simulink library "NeuroMuscularLibrary"  (R2019b)
settings: Solver=ode45  StartTime=0.0  StopTime=10.0  RelTol=1e-3  EnableMultiTasking=on
values from neighbouring files (symbols this model uses):
  a_18_19 = 116    [Prosthesis3R60Params.m]
  a_18_21 = 34    [Prosthesis3R60Params.m]
  a_2_3 = 18    [Prosthesis3R60Params.m]
  angle_offset = 0    [Prosthesis3R60Params.m]
  ankle_height = 0.08    [BodyMechParams.m]
  c = 0.05    [BodyMechParams.m]
  c_jointstop = 0.3 / (pi/180)    (= 17.1887338539)    [BodyMechParams.m]
  c_stance_comp_a0 = 885.0653    [Prosthesis3R60Params.m]
  c_stance_comp_a1 = 2.1443    [Prosthesis3R60Params.m]
  cg14 = 1/2*L14    (= 0.0475)    [Prosthesis3R60Params.m]
  cg25 = (5.45/11.05)*L25    (= 0.0379527149321)    [Prosthesis3R60Params.m]
  cg3 = (3.6/10.4)*L3    (= 0.0306346153846)    [Prosthesis3R60Params.m]
  d_fBall = 0.1    [BodyMechParams.m]
  d_fHeel = 0.05    [BodyMechParams.m]
  deltaLegAngleThr = 8*pi/180    (= 0.13962634016)    [CMGParams.m]
  DeltaThRef = 2e-3    (= 0.002)    [BodyMechParams.m]
  dt_visual = 0.001    [Prosthesis3R60Params.m]
  eref = 0.04    [BodyMechParams.m]
  Fmax = 4000    [MuscleEnergyTest.m]
  FmaxGLU = 1500    [BodyMechParams.m]
  footBallToAnkleDist = 0.16    [BodyMechParams.m]
  footBallToCenterDist = footLength/2    (= 0.1)    [BodyMechParams.m]
  footBallToHeelDist = footLength    (= 0.2)    [BodyMechParams.m]
  footCenterToCGDist = 0.14 - footBallToCenterDist    (= 0.04)    [BodyMechParams.m]
  footInertia = 0.005    [BodyMechParams.m]
  footLength = 0.2    [BodyMechParams.m]
  footMass = 1.25    [BodyMechParams.m]
  FT = 20    [MuscleEnergyTest.m]
  FT_GLU = 47.6    [BodyMechParams.m]
  g = 9.80665    [BodyMechParams.m]
  groundTheta = [atan(diff(groundZ)./diff(groundX)), 0]    [generateGround.m]
  groundZ = groundZ * stepSize/(largestStep+eps)    [generateGround.m]
  hatCenterToCGDist = 0.35 - hatHipToCenterDistLen    (= -0.05)    [BodyMechParams.m]
  hatHipToCenterDistLen = hatLength/2    (= 0.4)    [BodyMechParams.m]
  hatInertia = 3    [BodyMechParams.m]
  hatLeftHipToCenterDistWidth = .15    (= 0.15)    [BodyMechParams.m]
  hatLength = 0.8    [BodyMechParams.m]
  hatMass = 53.5    [BodyMechParams.m]
  hatThickness = 0.2    [BodyMechParams.m]
  hatWidth = 0.4    [BodyMechParams.m]
  J1011 = (4130)*1e-9    (= 4.13e-06)    [Prosthesis3R60Params.m]
  J1415 = (1.18*1e5)*1e-9    (= 0.000118)    [Prosthesis3R60Params.m]
  J18192021 = (6.86*1e4)*1e-9    (= 6.86e-05)    [Prosthesis3R60Params.m]
  J2526 = (3.59*1e4)*1e-9    (= 3.59e-05)    [Prosthesis3R60Params.m]
  J3467 = (25.96*1e4)*1e-9    (= 0.0002596)    [Prosthesis3R60Params.m]
  K = 5    [BodyMechParams.m]
  k_gn = k_gn/2    (= 39226.6)    [BodyMechParams.m]
  k_gt = k_gt/2    (= 39226.6)    [BodyMechParams.m]
  k_pressure = hatMass * g / DeltaThRef    (= 262327.8875)    [BodyMechParams.m]
  k_stance = 130000    [Prosthesis3R60Params.m]
  k_swing = 18750    [Prosthesis3R60Params.m]
  L0_stance = 0.08925    [Prosthesis3R60Params.m]
  L0_swing = 0.0896    [Prosthesis3R60Params.m]
  L10 = 7.9*1e-3    (= 0.0079)    [Prosthesis3R60Params.m]
  L11 = 3.3*1e-3    (= 0.0033)    [Prosthesis3R60Params.m]
  L14 = 95*1e-3    (= 0.095)    [Prosthesis3R60Params.m]
  L15 = 8.2*1e-3    (= 0.0082)    [Prosthesis3R60Params.m]
  L18 = 25.1*1e-3    (= 0.0251)    [Prosthesis3R60Params.m]
  L19 = 17.7*1e-3    (= 0.0177)    [Prosthesis3R60Params.m]
  L20 = 26*1e-3    (= 0.026)    [Prosthesis3R60Params.m]
  L21 = 1.7*1e-3    (= 0.0017)    [Prosthesis3R60Params.m]
  L25 = 76.95*1e-3    (= 0.07695)    [Prosthesis3R60Params.m]
  L26 = 2.8*1e-3    (= 0.0028)    [Prosthesis3R60Params.m]
  L3 = 88.5*1e-3    (= 0.0885)    [Prosthesis3R60Params.m]
  L4 = 1.7*1e-3    (= 0.0017)    [Prosthesis3R60Params.m]
  L6 = 40.25*1e-3    (= 0.04025)    [Prosthesis3R60Params.m]
  L7 = 14.9*1e-3    (= 0.0149)    [Prosthesis3R60Params.m]
  leg_l = [(thighLength - ankle_height/2) (shankLength - ankle_height/2)]    [BodyMechParams.m]
  legAngleSpeedMax = 10    [CMGParams.m]
  lopt = 0.055    [MuscleEnergyTest.m]
  loptBFSH = 0.12    [BodyMechParams.m]
  loptGAS = 0.05    [BodyMechParams.m]
  loptGLU = 0.11    [BodyMechParams.m]
  loptHAB = 0.09    [BodyMechParams.m]
  loptHAD = 0.10    (= 0.1)    [BodyMechParams.m]
  loptHAM = 0.10    (= 0.1)    [BodyMechParams.m]
  loptHFL = 0.11    [BodyMechParams.m]
  loptRF = 0.08    [BodyMechParams.m]
  loptSOL = 0.04    [BodyMechParams.m]
  loptTA = 0.06    [BodyMechParams.m]
  loptVAS = 0.08    [BodyMechParams.m]
  lslack = 0.245    [MuscleEnergyTest.m]
  lslackBFSH = 0.10    (= 0.1)    [BodyMechParams.m]
  lslackGAS = 0.40    (= 0.4)    [BodyMechParams.m]
  lslackGLU = 0.13    [BodyMechParams.m]
  lslackHAB = 0.07    [BodyMechParams.m]
  lslackHAD = 0.18    [BodyMechParams.m]
  lslackHAM = 0.31    [BodyMechParams.m]
  lslackHFL = 0.10    (= 0.1)    [BodyMechParams.m]
  lslackRF = 0.35    [BodyMechParams.m]
  lslackSOL = 0.26    [BodyMechParams.m]
  lslackTA = 0.24    [BodyMechParams.m]
  lslackVAS = 0.23    [BodyMechParams.m]
  m1011 = 49.5*1e-3    (= 0.0495)    [Prosthesis3R60Params.m]
  m1415 = 123.8*1e-3    (= 0.1238)    [Prosthesis3R60Params.m]
  m18192021 = 196.6*1e-3    (= 0.1966)    [Prosthesis3R60Params.m]
  m2526 = 58.3*1e-3    (= 0.0583)    [Prosthesis3R60Params.m]
  m3467 = 253.3*1e-3    (= 0.2533)    [Prosthesis3R60Params.m]
  mu_slide = 0.8    [BodyMechParams.m]
  mu_stick = 0.9    [BodyMechParams.m]
  N = 1.5    [BodyMechParams.m]    (also in cmaes.m = size(x,1); mergeCompareEnergyCosts.m = {S.name})
  phiKneeUpLimit = 5*pi/180    (= 0.0872664625997)    [BodyMechParams.m]
  phimaxGASa = (100-90)*pi/180    (= 0.174532925199)    [BodyMechParams.m]
  phimaxGASk = (180-140)*pi/180    (= 0.698131700798)    [BodyMechParams.m]
  phimaxRFk = (180-165)*pi/180    (= 0.261799387799)    [BodyMechParams.m]
  phimaxSOL = (100-90)*pi/180    (= 0.174532925199)    [BodyMechParams.m]
  phimaxTA = (80-90)*pi/180    (= -0.174532925199)    [BodyMechParams.m]
  phimaxVAS = (180-165)*pi/180    (= 0.261799387799)    [BodyMechParams.m]
  phirefBFSH = (180-160)*pi/180    (= 0.349065850399)    [BodyMechParams.m]
  phirefGASa = (80-90)*pi/180    (= -0.174532925199)    [BodyMechParams.m]
  phirefGASk = (180-165)*pi/180    (= 0.261799387799)    [BodyMechParams.m]
  phirefGLU = (120-180)*pi/180    (= -1.0471975512)    [BodyMechParams.m]
  phirefHAB = 10*pi/180    (= 0.174532925199)    [BodyMechParams.m]
  phirefHAD = 15*pi/180    (= 0.261799387799)    [BodyMechParams.m]
  phirefHAMh = (150-180)*pi/180    (= -0.523598775598)    [BodyMechParams.m]
  phirefHAMk = (180-180)*pi/180    (= 0)    [BodyMechParams.m]
  phirefHFL = (160-180)*pi/180    (= -0.349065850399)    [BodyMechParams.m]
  phirefRFh = (170-180)*pi/180    (= -0.174532925199)    [BodyMechParams.m]
  phirefRFk = (180-125)*pi/180    (= 0.959931088597)    [BodyMechParams.m]
  phirefSOL = (90-90)*pi/180    (= 0)    [BodyMechParams.m]
  ... (+64 more)
undefined symbols (not defined in the file or in its folder): ankleBackDriveGain, ankleCJointstop, ankleDgain, ankleFilterPID, ankleFilterSEA, ankleGearEff, ankleGearRatio, ankleIgain, ankleInitialAngle, ankleInputMass, ankleIntCoulomb, ankleIntDamping, ankleIntStatic, ankleParallelSpringDamping, ankleParallelSpringOffset, ankleParallelSpringStiffness, anklePgain, anklePlantarLimit, ankleSEADamping, ankleSEAStiffness, ankleTendonMass, ankleWMaxJointstop, D12_F, D12_S, D12_T, D12z_T, D13_F, D1G_F, D1G_HAT, D1G_S, D1G_T, D1Gy_F, DeltaS, DeltaSGLU, DeltaSHFL, dryFrictionDamping, dryFrictionStiffness, dryFrictionVelThresh, footMassp, FourBarL1, FourBarL3, GainDphiHATGLUst, GainDphiHATHABst, GainDphiHATHADst, GainDphiHATHFLst, GainFGASst, GainFGLUst, GainFHABst, GainFHAMst, GainFSOLst, GainFSOLTAst, GainFVASst, GainGAS, GainGLU, GainGLUswing, GainHAM, GainHAMHFL ... (+194)
libraries: sm_lib x332, nesl_utility x156, simulink x33, dspswit3 x30, $bdroot x19, simulink_extras x7
(part 1 of 15)
settings Model: Creator=nitisht  LastModifiedBy=Nathan
settings DataIOCC: LimitDataPoints=on  SaveFormat=Array  ReturnWorkspaceOutputs=off
settings OptimizationCC: LifeSpan=inf
settings DebuggingCC: UnderspecifiedInitializationDetection=Classic  MergeDetectMultiDrivingBlocksExec=none  SolverPrmCheckMsg=warning  StateNameClashWarn=warning  SFUnexpectedBacktrackingDiag=warning  SFNoUnconditionalDefaultTransitionDiag=warning  SFExecutionAtInitializationDiag=none  ArithmeticOperatorsInVariantConditions=warning
settings HardwareCC: ProdBitPerLong=64  ProdLargestAtomicFloat=None  ProdIntDivRoundTo=Undefined  ProdEndianess=Unspecified  ProdHWDeviceType=Intel->x86-64
settings ModelReferenceCC: PropagateSignalLabelsOutOfModel=off
settings SFSimCC: SimUseLocalCustomCode=off  CustomCodeUndefinedFunction=UseInterfaceOnly
settings RTWCC: RTWUseLocalCustomCode=off  RTWCompilerOptimization=on
settings CodeAppCC: StateflowObjectComments=on
settings GRTTargetCC: TargetLangStandard=C89/C90 (ANSI)  GeneratePreprocessorConditionals=Disable all
settings ConfigComp: CovMetricSettings=dw  CovHtmlReporting=on  CovSaveCumulativeToWorkspaceVar=on  CovSaveSingleToWorkspaceVar=on  CovExternalEMLEnable=off  CovSFcnEnable=off

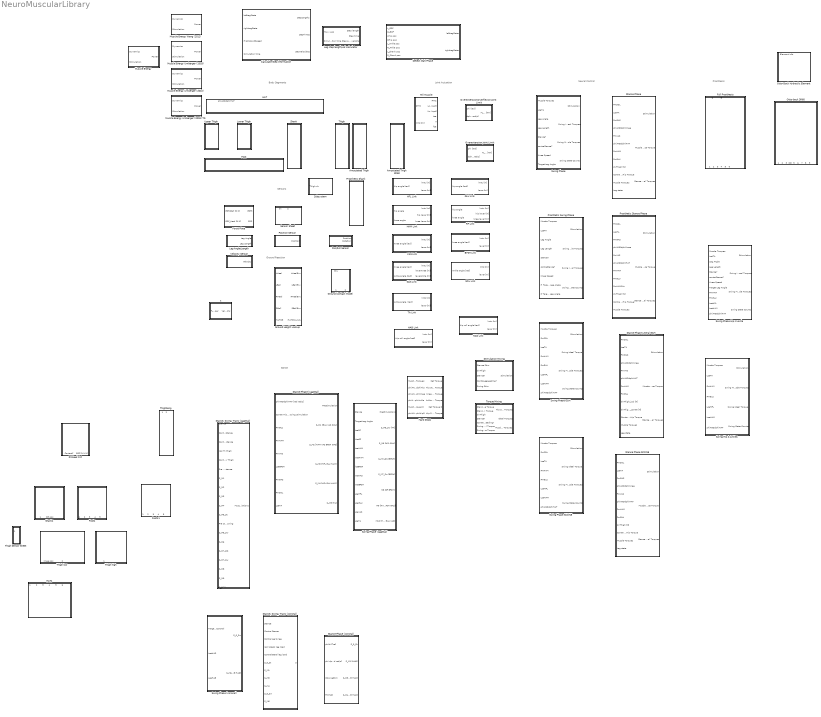
== system NeuroMuscularLibrary ==
  note: Body Segments
  note: Joint Actuation
  note: Sensors
  note: Ground Reaction
  note: Neural Control
  note: Prosthesis
  note: SONG
  Amputated Thigh : Subsystem
  Amputated Thigh 3R60 : Subsystem
  BFSH Link : Subsystem
  Calculate Step information : Subsystem
  Detect Gait Phase : Subsystem
  Foot : Subsystem
  Foots : Subsystem
  Foots1 : Subsystem
  Force Plate : Subsystem  TreatAsAtomicUnit=on
  Full Prosthesis : Subsystem
  GAS Link : Subsystem
  GLU Link : Subsystem
  Ground Contact Model : Subsystem
  Ground Height Lookup : Subsystem
  HAB Link : Subsystem
  HAD Link : Subsystem
  HAM Link : Subsystem
  HAT : Subsystem
  HATs : Subsystem
  HFL Link : Subsystem
  Hard Stops : Subsystem
  Hill Muscle : Subsystem  mask(Hill Type Muscle){Fmax=Fmax, lopt=lopt, vmax=vmax, lslack=lslack}
      mask prompts: Fmax "Max Isometric Force [N]"; lopt "Optimal Length [m]"; vmax "Max Contraction Velocity [m/s]"; lslack "Slack Length [m]"
      mask help:
      | Hill Type Muscle Model. This dialog allows you to specify several muscle-specific parameters. The block also requires several parameters to be defined globally in the matlab workspace:
      |
      | Excitation-contraction coupling parameters:
      | preA: preactivation
      | tau:  delay time constant [s]
      |
      | Contractile element (CE) force-length relationship:
      | w: width [lopt]
      | c: remaining force at +/- width
      |
      | CE force-velocity parameters:
      | N: eccentric force enhancement [Fmax]
      | K: shape factor
      |
      | Series elastic element (SE) force-length relationship
      | eref: tendon reference strain [lslack]
  Leg Angle/Length : Subsystem
  Leg step length/vel calculator : Subsystem
  Lower Thigh : Subsystem
  Muscle Energy : Subsystem  mask{lopt=loptGLU, FT=FT_GLU, Fmax=FmaxGLU, vmax=vmaxGLU}
      mask prompts: lopt "Optimum Length:"; FT "Percent Fast Twitch"; Fmax "Max Iso Force"; vmax "Max Contraction Velocity in m/s"
  Muscle Energy Umberger (2003) : Subsystem  mask{lopt=lopt, FT=FT, Fmax=Fmax, vmax=vmax}
      mask prompts: lopt "Optimum Length:"; FT "Percent Fast Twitch"; Fmax "Max Iso Force"; vmax "Max Contraction Velocity in m/s"
  Muscle Energy Umberger (2003) TG : Subsystem  mask{lopt=loptGLU, FT=FT_GLU, Fmax=FmaxGLU}
      mask prompts: lopt "Optimum Length:"; FT "Percent Fast Twitch"; Fmax "Max Iso Force"
  Muscle Energy Umberger (2010) : Subsystem  mask{lopt=lopt, FT=FT, Fmax=Fmax, vmax=vmax}
      mask prompts: lopt "Optimum Length:"; FT "Percent Fast Twitch"; Fmax "Max Iso Force"; vmax "Max Contraction Velocity in m/s"
  Muscle Energy Wang (2012) : Subsystem  mask{lopt=lopt, FT=FT, Fmax=Fmax}
      mask prompts: lopt "Optimum Length:"; FT "Percent Fast Twitch"; Fmax "Max Iso Force"
  Otto-Bock Hydraulic Element : Subsystem  mask{L0=0, k=0, Fd=0, dx_points=0, c_comp_a0=0, c_comp_a1=0, c_ext_a0=0, c_ext_a1=0, c=0}
      mask prompts: L0 "Slack length in m"; k "Stiffness in N/m"; Fd "Damping force look-up table"; dx_points "Velocity points look-up table"; c_comp_a0 "Compression damping coefficient a0"; c_comp_a1 "Compression damping coefficient a1"; c_ext_a0 "Extension damping coefficient a0"; c_ext_a1 "Extension damping coefficient a1"; c "Damping coefficient look-up table"
  Otto-bock 3R60 : Subsystem
  Overextension Joint Limit : Subsystem  mask{phiUpLimit=phiKneeUpLimit, ext=1}
      mask prompts: phiUpLimit "Upper Limit [rad]"; ext "Extension values are positive or negative?"
      mask help:
      | This block implements a hard joint limit that will prevent the joint from extending past the specified upper limit.
      |
      | Used for the knee and hip joints.
  Overextension/Overflexion Joint Limit : Subsystem  mask(Overextension/Overflexion Joint Limit){phiUpLimit=0, phiLowLimit=0}
      mask prompts: phiUpLimit "Upper Limit [rad]"; phiLowLimit "Lower Limit [rad]"
      mask help:
      | This block implents a hard joint limit that will prevent the joint from overextending past the specified upper limit and overflexing below the lower limit.
      |
      | Used for the Ankle Joint.
  Pos/Rot Sensor : Subsystem
  Position Sensor : Subsystem
  Prosthetic Shank : Subsystem
  Prosthetic Stance Phase : Subsystem  mask{GainHAM=RGainHAM, GainHAMCut=RGainHAMCut, GainGLU=RGainGLU, GainSOL=RGainSOL, GainSOLTA=RGainSOLTA, GainTA=RGainTA, GainGAS=RGainGAS, GainVAS=RGainVAS, GainKneeOverExt=RGainKneeOverExt, PosGainGG=RPosGainGG, SpeedGainGG=RSpeedGainGG, Kglu=RKglu}
  Prosthetic Swing Phase : Subsystem  mask{GainTA=RGainTA, hipPGain=RhipPGain, hipDGain=RhipDGain, legAngleFilter=RlegAngleFilter, kneeFlexGain=RkneeFlexGain, kneeHoldGain1=RkneeHoldGain1, kneeHoldGain2=RkneeHoldGain2, kneeStopGain=RkneeStopGain, kneeExtendGain=RkneeExtendGain, legLengthClr=RlegLengthClr}
  RF Link : Subsystem
  RMHeel Cnt : Subsystem
  SOL Link : Subsystem
  Sensor Sheet : Subsystem
  Shank : Subsystem
  Shanks : Subsystem
  Stance Phase : Subsystem  mask{GainHAM=GainHAM, GainGLU=GainGLU, GainSOL=GainSOL, GainSOLTA=GainSOLTA, GainTA=GainTA, GainGAS=GainGAS, GainVAS=GainVAS, GainKneeOverExt=GainKneeOverExt, PosGainGG=PosGainGG, SpeedGainGG=SpeedGainGG, Kglu=Kglu, PreStimSOL=PreStimSOL, PreStimTA=PreStimTA, PreStimGAS=PreStimGAS, PreStimVAS=PreStimVAS, PreStimGLU=PreStimGLU, PreStimHAM=PreStimHAM, PreStimHFL=PreStimHFL, DeltaS=0}
  Stance Phase (coronal) : Subsystem  TreatAsAtomicUnit=on
  Stance Phase (sagittal) : Subsystem  TreatAsAtomicUnit=on
  Stance Phase Literal G&H : Subsystem  mask{GainHAM=GainHAM, GainGLU=GainGLU, GainSOL=GainSOL, GainSOLTA=GainSOLTA, GainTA=GainTA, GainGAS=GainGAS, GainVAS=GainVAS, GainKneeOverExt=GainKneeOverExt, PosGainGG=PosGainGG, SpeedGainGG=SpeedGainGG, Kglu=Kglu, Kbw=Kbw, DeltaS=DeltaS}
  Stance Phase SCONE : Subsystem  mask{GainHAM=GainHAM, GainGLU=GainGLU, GainSOL=GainSOL, GainSOLTA=GainSOLTA, GainTA=GainTA, GainGAS=GainGAS, GainVAS=GainVAS, GainKneeOverExt=GainKneeOverExt, PosGainGG=PosGainGG, SpeedGainGG=SpeedGainGG, Kglu=Kglu, Kham=Kham, Khfl=Khfl, DeltaSGLU=DeltaSGLU, DeltaSHFL=DeltaSHFL}
  "Stance, Swing, Trans (coronal)" : Subsystem  TreatAsAtomicUnit=on
  "Stance, Swing, Trans (sagittal)" : Subsystem
  Stimulation Mixing : Subsystem
  Subsystem : Subsystem
  Swing Hip & Ankles : Subsystem  mask{GainTA=GainTAswing, GainHAM=GainHAMswing, GainGLU=GainGLUswing, GainHFL=GainHFL, GainHAMHFL=GainHAMHFL, Klean=Klean, PreStimSOL=PreStimSOLswing, PreStimTA=PreStimTAswing, PreStimGAS=PreStimGASswing, PreStimVAS=PreStimVASswing, PreStimGLU=PreStimGLUswing, PreStimHAM=PreStimHAMswing, PreStimHFL=PreStimHFLswing}
  Swing Phase : Subsystem  mask{GainTA=GainTA, hipPGain=hipPGain, hipDGain=hipDGain, legAngleFilter=legAngleFilter, kneeFlexGain=kneeFlexGain, kneeHoldGain1=kneeHoldGain1, kneeHoldGain2=kneeHoldGain2, kneeStopGain=kneeStopGain, kneeExtendGain=kneeExtendGain, legLengthClr=legLengthClr}
  Swing Phase (coronal) : Subsystem  TreatAsAtomicUnit=on
  Swing Phase (sagittal) : Subsystem  TreatAsAtomicUnit=on
  Swing Phase G&H : Subsystem  mask{GainTA=GainTA, GainHAM=GainHAM, GainGLU=GainGLU, GainHFL=GainHFL, GainHAMHFL=GainHAMHFL, Klean=Klean}
  Swing Phase Hip muscle : Subsystem  mask{GainTA=GainTA, hipPGain=hipPGain, hipDGain=hipDGain, legAngleFilter=legAngleFilter, kneeFlexGain=kneeFlexGain, kneeHoldGain1=kneeHoldGain1, kneeHoldGain2=kneeHoldGain2, kneeStopGain=kneeStopGain, kneeExtendGain=kneeExtendGain, legLengthClr=legLengthClr}
  Swing Phase SCONE : Subsystem  mask{GainTA=GainTA, GainHAM=GainHAM, GainGLU=GainGLU, GainHFL=GainHFL, GainHAMHFL=GainHAMHFL, Klean=Klean}
  TA Link : Subsystem
  Thigh : Subsystem
  Thigh Sensor Sheet : Subsystem
  Thigh high : Subsystem
  Thigh low : Subsystem
  ThighSong : Subsystem
  Torque Mixing : Subsystem
  Upper Thigh : Subsystem
  VAS Link : Subsystem
  Velocity Sensor : Subsystem
  c : Subsystem  mask{a0=c_stance_comp_a0, a1=c_stance_comp_a1}
      mask prompts: a0 "Value of a0"; a1 "Value of a1"

== system NeuroMuscularLibrary/Amputated Thigh ==
  Knee to Center : sm_lib/Frames and Transforms/Rigid Transform  TranslationMethod=Cartesian  TranslationStandardOffset=0  TranslationLengthUnit=m  TranslationStandardAxis=+Z  TranslationCartesianOffset=[0 thighKneeToCenterDist 0]  TranslationROffset=0  TranslationROffsetUnits=m  TranslationZOffset=0  TranslationZOffsetUnits=m  TranslationThetaOffset=0  TranslationThetaOffsetUnits=deg  RotationMethod=AlignedAxes  RotationAngleUnits=deg  RotationStandardAxis=+Z  RotationAngle=0  RotationArbitraryAxis=[0 0 1]  FollAlignAxisA=+Z  BaseAlignAxisA=+Y  FollAlignAxisB=+X  BaseAlignAxisB=+X  RotationSequenceAxes=FollowerAxes  RotationSequence=XYX  RotationSequenceAngles=[0 0 0]  RotationSequenceAnglesUnits=deg  RotationMatrix=[1 0 0; 0 1 0; 0 0 1]
  Knee to Center1 : sm_lib/Frames and Transforms/Rigid Transform  TranslationMethod=Cartesian  TranslationStandardOffset=0  TranslationLengthUnit=m  TranslationStandardAxis=+Z  TranslationCartesianOffset=[0 0 .05]  TranslationROffset=0  TranslationROffsetUnits=m  TranslationZOffset=0  TranslationZOffsetUnits=m  TranslationThetaOffset=0  TranslationThetaOffsetUnits=deg  RotationMethod=None  RotationAngleUnits=deg  RotationStandardAxis=+Z  RotationAngle=0  RotationArbitraryAxis=[0 0 1]  FollAlignAxisA=+Z  BaseAlignAxisA=+Y  FollAlignAxisB=+X  BaseAlignAxisB=+X  RotationSequenceAxes=FollowerAxes  RotationSequence=XYX  RotationSequenceAngles=[0 0 0]  RotationSequenceAnglesUnits=deg  RotationMatrix=[1 0 0; 0 1 0; 0 0 1]
  Knee to Sensor Sheet : sm_lib/Frames and Transforms/Rigid Transform  TranslationMethod=Cartesian  TranslationStandardOffset=0  TranslationLengthUnit=m  TranslationStandardAxis=+Z  TranslationCartesianOffset=[0 thighKneeToHipDist 0]  TranslationROffset=0  TranslationROffsetUnits=m  TranslationZOffset=0  TranslationZOffsetUnits=m  TranslationThetaOffset=0  TranslationThetaOffsetUnits=deg  RotationMethod=None  RotationAngleUnits=deg  RotationStandardAxis=+Z  RotationAngle=0  RotationArbitraryAxis=[0 0 1]  FollAlignAxisA=+Z  BaseAlignAxisA=+X  FollAlignAxisB=+Y  BaseAlignAxisB=+Y  RotationSequenceAxes=FollowerAxes  RotationSequence=XYX  RotationSequenceAngles=[0 0 0]  RotationSequenceAnglesUnits=deg  RotationMatrix=[1 0 0; 0 1 0; 0 0 1]
  Thigh CG : sm_lib/Frames and Transforms/Reference Frame
  Thigh Center to CG : sm_lib/Frames and Transforms/Rigid Transform  TranslationMethod=Cartesian  TranslationStandardOffset=0  TranslationLengthUnit=m  TranslationStandardAxis=+Z  TranslationCartesianOffset=[0 0 thighCenterToCGDist]  TranslationROffset=0  TranslationROffsetUnits=m  TranslationZOffset=0  TranslationZOffsetUnits=m  TranslationThetaOffset=0  TranslationThetaOffsetUnits=deg  RotationMethod=None  RotationAngleUnits=deg  RotationStandardAxis=+Z  RotationAngle=0  RotationArbitraryAxis=[0 0 1]  FollAlignAxisA=+X  BaseAlignAxisA=+Y  FollAlignAxisB=+Y  BaseAlignAxisB=+Z  RotationSequenceAxes=FollowerAxes  RotationSequence=XYX  RotationSequenceAngles=[0 0 0]  RotationSequenceAnglesUnits=deg  RotationMatrix=[1 0 0; 0 1 0; 0 0 1]
  Thigh Graphic : sm_lib/Body Elements/Cylindrical Solid  GraphicAmbientColor=[0.15 0.15 0.15 1.0]  BasedOnType=Density  CenterOfMass=[0 0 thighCenterToCGDist]  CenterOfMassUnits=m  GraphicDiffuseColor=[0.5 0.5 0.5]  CylinderLength=thighLength-.1  CylinderLengthUnits=m  CylinderRadius=.075  CylinderRadiusUnits=m  Density=1000  DensityUnits=kg/(m^3)  DoExposeReferenceFrame=on  GraphicEmissiveColor=[0.0 0.0 0.0 1.0]  ExportEntireGeometry=off  SerializedFrames=<Frames/>  MarkerShape=Sphere  MarkerSize=10  GraphicType=FromGeometry  InertiaType=PointMass  Mass=0  MassUnits=kg  MomentsOfInertia=[thighInertia 0 0]  MomentsOfInertiaUnits=kg*m^2  GraphicOpacity=1.0  ProductsOfInertia=[0 0 0]  ProductsOfInertiaUnits=kg*m^2  GraphicShininess=75  GraphicSpecularColor=[0.5 0.5 0.5 1.0]  GraphicVisPropType=SimpleVisualProperties
  Thigh inertia : sm_lib/Body Elements/Cylindrical Solid  GraphicAmbientColor=[0.15 0.15 0.15 1.0]  BasedOnType=Density  CenterOfMass=[0 0 thighCenterToCGDist]  CenterOfMassUnits=m  GraphicDiffuseColor=[0.5 0.5 0.5]  CylinderLength=thighLength  CylinderLengthUnits=m  CylinderRadius=.075  CylinderRadiusUnits=m  Density=1000  DensityUnits=kg/(m^3)  DoExposeReferenceFrame=on  GraphicEmissiveColor=[0.0 0.0 0.0 1.0]  ExportEntireGeometry=off  SerializedFrames=<Frames/>  MarkerShape=Sphere  MarkerSize=10  GraphicType=None  InertiaType=Custom  Mass=thighMass  MassUnits=kg  MomentsOfInertia=[thighInertia 0 0]  MomentsOfInertiaUnits=kg*m^2  GraphicOpacity=1.0  ProductsOfInertia=[0 0 0]  ProductsOfInertiaUnits=kg*m^2  GraphicShininess=75  GraphicSpecularColor=[0.5 0.5 0.5 1.0]  GraphicVisPropType=SimpleVisualProperties
  Knee : PMIOPort  Side=Left
  Sensor Sheet : PMIOPort  Port=2  Side=Right
  connections:
  Knee/RConn1 -- Knee to Center/LConn1 -- Knee to Sensor Sheet/LConn1
  Knee to Center/RConn1 -- Knee to Center1/LConn1 -- Thigh inertia/RConn1 -- Thigh Center to CG/LConn1
  Knee to Sensor Sheet/RConn1 -- Sensor Sheet/RConn1
  Thigh Center to CG/RConn1 -- Thigh CG/RConn1
  Thigh Graphic/RConn1 -- Knee to Center1/RConn1

== system NeuroMuscularLibrary/Amputated Thigh 3R60 ==
  Knee to Center : sm_lib/Frames and Transforms/Rigid Transform  TranslationMethod=Cartesian  TranslationStandardOffset=0  TranslationLengthUnit=m  TranslationStandardAxis=+Z  TranslationCartesianOffset=[0 thighKneeToCenterDist-0.1 0]  TranslationROffset=0  TranslationROffsetUnits=m  TranslationZOffset=0  TranslationZOffsetUnits=m  TranslationThetaOffset=0  TranslationThetaOffsetUnits=deg  RotationMethod=AlignedAxes  RotationAngleUnits=deg  RotationStandardAxis=+Z  RotationAngle=0  RotationArbitraryAxis=[0 0 1]  FollAlignAxisA=+Z  BaseAlignAxisA=+Y  FollAlignAxisB=+X  BaseAlignAxisB=+X  RotationSequenceAxes=FollowerAxes  RotationSequence=XYX  RotationSequenceAngles=[0 0 0]  RotationSequenceAnglesUnits=deg  RotationMatrix=[1 0 0; 0 1 0; 0 0 1]
  Knee to Center1 : sm_lib/Frames and Transforms/Rigid Transform  TranslationMethod=Cartesian  TranslationStandardOffset=0  TranslationLengthUnit=m  TranslationStandardAxis=+Z  TranslationCartesianOffset=[0 0 .05]  TranslationROffset=0  TranslationROffsetUnits=m  TranslationZOffset=0  TranslationZOffsetUnits=m  TranslationThetaOffset=0  TranslationThetaOffsetUnits=deg  RotationMethod=None  RotationAngleUnits=deg  RotationStandardAxis=+Z  RotationAngle=0  RotationArbitraryAxis=[0 0 1]  FollAlignAxisA=+Z  BaseAlignAxisA=+Y  FollAlignAxisB=+X  BaseAlignAxisB=+X  RotationSequenceAxes=FollowerAxes  RotationSequence=XYX  RotationSequenceAngles=[0 0 0]  RotationSequenceAnglesUnits=deg  RotationMatrix=[1 0 0; 0 1 0; 0 0 1]
  Knee to Sensor Sheet : sm_lib/Frames and Transforms/Rigid Transform  TranslationMethod=Cartesian  TranslationStandardOffset=0  TranslationLengthUnit=m  TranslationStandardAxis=+Z  TranslationCartesianOffset=[0 thighKneeToHipDist-0.1 0]  TranslationROffset=0  TranslationROffsetUnits=m  TranslationZOffset=0  TranslationZOffsetUnits=m  TranslationThetaOffset=0  TranslationThetaOffsetUnits=deg  RotationMethod=None  RotationAngleUnits=deg  RotationStandardAxis=+Z  RotationAngle=0  RotationArbitraryAxis=[0 0 1]  FollAlignAxisA=+Z  BaseAlignAxisA=+X  FollAlignAxisB=+Y  BaseAlignAxisB=+Y  RotationSequenceAxes=FollowerAxes  RotationSequence=XYX  RotationSequenceAngles=[0 0 0]  RotationSequenceAnglesUnits=deg  RotationMatrix=[1 0 0; 0 1 0; 0 0 1]
  Thigh CG : sm_lib/Frames and Transforms/Reference Frame
  Thigh Center to CG : sm_lib/Frames and Transforms/Rigid Transform  TranslationMethod=Cartesian  TranslationStandardOffset=0  TranslationLengthUnit=m  TranslationStandardAxis=+Z  TranslationCartesianOffset=[0 0 thighCenterToCGDist]  TranslationROffset=0  TranslationROffsetUnits=m  TranslationZOffset=0  TranslationZOffsetUnits=m  TranslationThetaOffset=0  TranslationThetaOffsetUnits=deg  RotationMethod=None  RotationAngleUnits=deg  RotationStandardAxis=+Z  RotationAngle=0  RotationArbitraryAxis=[0 0 1]  FollAlignAxisA=+X  BaseAlignAxisA=+Y  FollAlignAxisB=+Y  BaseAlignAxisB=+Z  RotationSequenceAxes=FollowerAxes  RotationSequence=XYX  RotationSequenceAngles=[0 0 0]  RotationSequenceAnglesUnits=deg  RotationMatrix=[1 0 0; 0 1 0; 0 0 1]
  Thigh Graphic : sm_lib/Body Elements/Cylindrical Solid  GraphicAmbientColor=[0.15 0.15 0.15 1.0]  BasedOnType=Density  CenterOfMass=[0 0 thighCenterToCGDist]  CenterOfMassUnits=m  GraphicDiffuseColor=[0.5 0.5 0.5]  CylinderLength=thighLength-.1  CylinderLengthUnits=m  CylinderRadius=.075  CylinderRadiusUnits=m  Density=1000  DensityUnits=kg/(m^3)  DoExposeReferenceFrame=on  GraphicEmissiveColor=[0.0 0.0 0.0 1.0]  ExportEntireGeometry=off  SerializedFrames=<Frames/>  MarkerShape=Sphere  MarkerSize=10  GraphicType=FromGeometry  InertiaType=PointMass  Mass=0  MassUnits=kg  MomentsOfInertia=[thighInertia 0 0]  MomentsOfInertiaUnits=kg*m^2  GraphicOpacity=1.0  ProductsOfInertia=[0 0 0]  ProductsOfInertiaUnits=kg*m^2  GraphicShininess=75  GraphicSpecularColor=[0.5 0.5 0.5 1.0]  GraphicVisPropType=SimpleVisualProperties
  Thigh inertia : sm_lib/Body Elements/Cylindrical Solid  GraphicAmbientColor=[0.15 0.15 0.15 1.0]  BasedOnType=Density  CenterOfMass=[0 0 thighCenterToCGDist]  CenterOfMassUnits=m  GraphicDiffuseColor=[0.5 0.5 0.5]  CylinderLength=thighLength  CylinderLengthUnits=m  CylinderRadius=.075  CylinderRadiusUnits=m  Density=1000  DensityUnits=kg/(m^3)  DoExposeReferenceFrame=on  GraphicEmissiveColor=[0.0 0.0 0.0 1.0]  ExportEntireGeometry=off  SerializedFrames=<Frames/>  MarkerShape=Sphere  MarkerSize=10  GraphicType=None  InertiaType=Custom  Mass=thighMass  MassUnits=kg  MomentsOfInertia=[thighInertia 0 0]  MomentsOfInertiaUnits=kg*m^2  GraphicOpacity=1.0  ProductsOfInertia=[0 0 0]  ProductsOfInertiaUnits=kg*m^2  GraphicShininess=75  GraphicSpecularColor=[0.5 0.5 0.5 1.0]  GraphicVisPropType=SimpleVisualProperties
  Knee : PMIOPort  Side=Left
  Sensor Sheet : PMIOPort  Port=2  Side=Right
  connections:
  Thigh Graphic/RConn1 -- Knee to Center1/RConn1
  Thigh Center to CG/RConn1 -- Thigh CG/RConn1
  Knee to Sensor Sheet/RConn1 -- Sensor Sheet/RConn1
  Thigh Center to CG/LConn1 -- Thigh inertia/RConn1 -- Knee to Center1/LConn1 -- Knee to Center/RConn1
  Knee to Sensor Sheet/LConn1 -- Knee to Center/LConn1 -- Knee/RConn1

== system NeuroMuscularLibrary/BFSH Link ==
  note: BFSH Attachment
  knee angle [rad] : Inport
  Constant : Constant  Value=lslackBFSH+loptBFSH
  Constant1 : Constant  Value=rBFSH
  Constant2 : Constant  Value=phirefBFSH
  Gain2 : Gain  Gain=rhoBFSH
  Multiply : Gain  Gain=-1
  Product : Product  RndMeth=Zero
  Sum2 : Sum  Inputs=|-+
  Sum5 : Sum  Inputs=|++
  lmtu [m] : Outport
  lever [m] : Outport  Port=2
  wires:
  Sum2/1 -> Multiply/1
  Constant1/1 -> Product/2, lever [m]/1
  Constant/1 -> Sum5/1
  Constant2/1 -> Sum2/2
  Sum5/1 -> lmtu [m]/1
  Gain2/1 -> Sum5/2
  Product/1 -> Gain2/1
  knee angle [rad]/1 -> Sum2/1
  Multiply/1 -> Product/1

== system NeuroMuscularLibrary/Calculate Step information ==
  leftLegState : Inport
  rightLegState : Inport  Port=2
  HipPosAndSpeed : Inport  Port=3
  Simulation time : Inport  Port=4
  Constant : Constant  Value=-4
  Constant1 : Constant  Value=-4
  Difference1 : simulink/Discrete/Difference  ICPrevInput=0.0  OutMin=[]  OutMax=[]  OutDataType=fixdt(1, 16)  OutScaling=2^-10  DoSatur=off
  Difference2 : simulink/Discrete/Difference  ICPrevInput=0.0  OutMin=[]  OutMax=[]  OutDataType=fixdt(1, 16)  OutScaling=2^-10  DoSatur=off
  Left Leg step length/vel calculator : $bdroot/Leg step length//vel calculator  SystemSampleTime=-1  Latency=0  AutoFrameSizeCalculation=off
  Mux : Mux  Inputs=2
  Mux2 : Mux  Inputs=2
  Mux3 : Mux  Inputs=2
  Relational Operator : RelationalOperator  Operator=<=  OutDataTypeStr=boolean  RndMeth=Simplest
  Relational Operator1 : RelationalOperator  Operator=<=  OutDataTypeStr=boolean  RndMeth=Simplest
  Right Leg step length/vel calculator : $bdroot/Leg step length//vel calculator  SystemSampleTime=-1  Latency=0  AutoFrameSizeCalculation=off
  Selector1 : Selector  InputPortWidth=3  IndexOptions=Index vector (dialog)  Indices=[1]  OutputSizes=1
  stepLengths : Outport
  stepTimes : Outport  Port=2
  stepVelocities : Outport  Port=3
  wires:
  Difference1/1 -> Relational Operator/1
  Constant/1 -> Relational Operator/2
  Right Leg step length/vel calculator/1 -> Mux/2  "right Leg step length"
  Left Leg step length/vel calculator/1 -> Mux/1  "left Leg step length"
  Simulation time/1 -> Right Leg step length/vel calculator/2, Left Leg step length/vel calculator/2
  Relational Operator/1 -> Left Leg step length/vel calculator/Enable
  Constant1/1 -> Relational Operator1/2
  Selector1/1 -> Right Leg step length/vel calculator/1, Left Leg step length/vel calculator/1
  Right Leg step length/vel calculator/3 -> Mux2/2  "right Leg step velocity"
  HipPosAndSpeed/1 -> Selector1/1
  Relational Operator1/1 -> Right Leg step length/vel calculator/Enable
  Mux2/1 -> stepVelocities/1
  Left Leg step length/vel calculator/3 -> Mux2/1  "left Leg step velocity"
  Right Leg step length/vel calculator/2 -> Mux3/2  "right Leg step time"
  Difference2/1 -> Relational Operator1/1
  Mux/1 -> stepLengths/1
  Left Leg step length/vel calculator/2 -> Mux3/1  "left Leg step time"
  Mux3/1 -> stepTimes/1
  rightLegState/1 -> Difference2/1
  leftLegState/1 -> Difference1/1

== system NeuroMuscularLibrary/Detect Gait Phase ==
  L_GRF : Inport
  R_GRF : Inport  Port=2
  LHip pos : Inport  Port=3
  RHip pos : Inport  Port=4
  L_Ankle pos : Inport  Port=5
  R_Ankle pos : Inport  Port=6
  L_Shank pos : Inport  Port=7
  R_Shank pos : Inport  Port=8
  Add : Sum  Inputs=+-
  Add1 : Sum  Inputs=-+
  Add2 : Sum  Inputs=+-
  Add3 : Sum  Inputs=+-
  Add4 : Sum
  Delay One Step : Delay  DelayLength=1
  Delay One Step1 : Delay  DelayLength=1
  Fcn : Fcn  Expr=sqrt( u(1)^2 + u(2)^2 + u(3)^2 )
  Fcn1 : Fcn  Expr=sqrt( u(1)^2 + u(2)^2 + u(3)^2 )
  MATLAB Function : MATLAB Function  TreatAsAtomicUnit=on
  Multiply : Gain  Gain=1/2
  Selector : Selector  InputPortWidth=3  IndexOptions=Index vector (dialog)  Indices=[1]  OutputSizes=1
  Selector1 : Selector  InputPortWidth=3  IndexOptions=Index vector (dialog)  Indices=[1]  OutputSizes=1
  Selector2 : Selector  InputPortWidth=3  IndexOptions=Index vector (dialog)  Indices=[2]  OutputSizes=1
  Selector3 : Selector  InputPortWidth=3  IndexOptions=Index vector (dialog)  Indices=[2]  OutputSizes=1
  leftLegState : Outport
  rightLegState : Outport  Port=2
  wires:
  MATLAB Function/2(rightLegState) -> Delay One Step1/1, rightLegState/1
  MATLAB Function/1(leftLegState) -> Delay One Step/1, leftLegState/1
  Delay One Step/1 -> MATLAB Function/1(leftLegState_old)
  Delay One Step1/1 -> MATLAB Function/2(rightLegState_old)
  L_GRF/1 -> Selector2/1
  R_GRF/1 -> Selector3/1
  L_Ankle pos/1 -> Add/1, Add2/1
  R_Ankle pos/1 -> Add1/2, Add3/1
  Add/1 -> Selector/1
  Selector/1 -> MATLAB Function/5(L_SAGGpos)  "x"
  Add1/1 -> Selector1/1
  Selector1/1 -> MATLAB Function/6(R_SAGGpos)  "x"
  L_Shank pos/1 -> Add2/2
  R_Shank pos/1 -> Add3/2
  Add3/1 -> Fcn/1
  Add2/1 -> Fcn1/1
  Fcn1/1 -> MATLAB Function/7(L_norm_foot_shank)
  Fcn/1 -> MATLAB Function/8(R_norm_foot_shank)
  Selector2/1 -> MATLAB Function/3(L_GRF)  "z"
  Selector3/1 -> MATLAB Function/4(R_GRF)  "z"
  Add4/1 -> Multiply/1
  Multiply/1 -> Add1/1, Add/2
  LHip pos/1 -> Add4/1
  RHip pos/1 -> Add4/2

== system NeuroMuscularLibrary/Foot ==
  Ball To Ankle : sm_lib/Frames and Transforms/Rigid Transform  TranslationMethod=Cartesian  TranslationStandardOffset=0  TranslationLengthUnit=m  TranslationStandardAxis=+Z  TranslationCartesianOffset=[-footBallToAnkleDist 0 0]  TranslationROffset=0  TranslationROffsetUnits=m  TranslationZOffset=0  TranslationZOffsetUnits=m  TranslationThetaOffset=0  TranslationThetaOffsetUnits=deg  RotationMethod=None  RotationAngleUnits=deg  RotationStandardAxis=+Z  RotationAngle=0  RotationArbitraryAxis=[0 0 1]  FollAlignAxisA=+X  BaseAlignAxisA=+Y  FollAlignAxisB=+Y  BaseAlignAxisB=+Z  RotationSequenceAxes=FollowerAxes  RotationSequence=XYX  RotationSequenceAngles=[0 0 0]  RotationSequenceAnglesUnits=deg  RotationMatrix=[1 0 0; 0 1 0; 0 0 1]
  Ball To Heel : sm_lib/Frames and Transforms/Rigid Transform  TranslationMethod=Cartesian  TranslationStandardOffset=0  TranslationLengthUnit=m  TranslationStandardAxis=+Z  TranslationCartesianOffset=[-footBallToHeelDist 0 0]  TranslationROffset=0  TranslationROffsetUnits=m  TranslationZOffset=0  TranslationZOffsetUnits=m  TranslationThetaOffset=0  TranslationThetaOffsetUnits=deg  RotationMethod=None  RotationAngleUnits=deg  RotationStandardAxis=+Z  RotationAngle=0  RotationArbitraryAxis=[0 0 1]  FollAlignAxisA=+X  BaseAlignAxisA=+Y  FollAlignAxisB=+Y  BaseAlignAxisB=+Z  RotationSequenceAxes=FollowerAxes  RotationSequence=XYX  RotationSequenceAngles=[0 0 0]  RotationSequenceAnglesUnits=deg  RotationMatrix=[1 0 0; 0 1 0; 0 0 1]
  Ball to Center : sm_lib/Frames and Transforms/Rigid Transform  TranslationMethod=Cartesian  TranslationStandardOffset=0  TranslationLengthUnit=m  TranslationStandardAxis=+Z  TranslationCartesianOffset=[-footBallToCenterDist .025 0]  TranslationROffset=0  TranslationROffsetUnits=m  TranslationZOffset=0  TranslationZOffsetUnits=m  TranslationThetaOffset=0  TranslationThetaOffsetUnits=deg  RotationMethod=None  RotationAngleUnits=deg  RotationStandardAxis=+Z  RotationAngle=0  RotationArbitraryAxis=[0 0 1]  FollAlignAxisA=+X  BaseAlignAxisA=+Y  FollAlignAxisB=+Y  BaseAlignAxisB=+Z  RotationSequenceAxes=FollowerAxes  RotationSequence=XYX  RotationSequenceAngles=[0 0 0]  RotationSequenceAnglesUnits=deg  RotationMatrix=[1 0 0; 0 1 0; 0 0 1]
  Foot Solid : sm_lib/Body Elements/Brick Solid  GraphicAmbientColor=[0.15 0.15 0.15 1.0]  BasedOnType=Density  BrickDimensions=[footLength .05 .1]  BrickDimensionUnits=m  CenterOfMass=[-footCenterToCGDist 0 0]  CenterOfMassUnits=m  GraphicDiffuseColor=[0.5 0.5 0.5]  Density=1000  DensityUnits=kg/(m^3)  DoExposeReferenceFrame=on  GraphicEmissiveColor=[0.0 0.0 0.0 1.0]  ExportEntireGeometry=off  SerializedFrames=<Frames/>  MarkerShape=Sphere  MarkerSize=10  GraphicType=FromGeometry  InertiaType=Custom  Mass=footMass  MassUnits=kg  MomentsOfInertia=[0 0 footInertia]  MomentsOfInertiaUnits=kg*m^2  GraphicOpacity=1.0  ProductsOfInertia=[0 0 0]  ProductsOfInertiaUnits=kg*m^2  GraphicShininess=75  GraphicSpecularColor=[0.5 0.5 0.5 1.0]  GraphicVisPropType=SimpleVisualProperties
  Ankle : PMIOPort  Side=Right
  Heel : PMIOPort  Port=2  Side=Left
  Ball : PMIOPort  Port=3  Side=Left
  connections:
  Ball To Heel/LConn1 -- Ball to Center/LConn1 -- Ball/RConn1 -- Ball To Ankle/LConn1
  Ball to Center/RConn1 -- Foot Solid/RConn1
  Ball To Ankle/RConn1 -- Ankle/RConn1
  Ball To Heel/RConn1 -- Heel/RConn1

== system NeuroMuscularLibrary/Foots ==
  Brick Solid : sm_lib/Body Elements/Brick Solid  GraphicAmbientColor=[0.15 0.15 0.15 1.0]  BasedOnType=Mass  BrickDimensions=[D13_F ankle_height d_fBall]  BrickDimensionUnits=m  CenterOfMass=[0 0 0]  CenterOfMassUnits=m  GraphicDiffuseColor=[0.5 0.5 0.5]  Density=0  DensityUnits=kg/m^3  DoExposeReferenceFrame=on  GraphicEmissiveColor=[0.0 0.0 0.0 1.0]  ExportEntireGeometry=off  SerializedFrames=<Frames/>  MarkerShape=Sphere  MarkerSize=10  GraphicType=FromGeometry  InertiaType=CalculateFromGeometry  Mass=0  MassUnits=kg  MomentsOfInertia=[1 1 1]  MomentsOfInertiaUnits=kg*m^2  GraphicOpacity=1.0  ProductsOfInertia=[0 0 0]  ProductsOfInertiaUnits=kg*m^2  GraphicShininess=75  GraphicSpecularColor=[0.5 0.5 0.5 1.0]  GraphicVisPropType=SimpleVisualProperties
  CS{1,5..6,9..10} (5 alike) : sm_lib/Frames and Transforms/Rigid Transform  TranslationMethod=None  TranslationStandardOffset=0  TranslationLengthUnit=m  TranslationStandardAxis=+Z  TranslationCartesianOffset=[0 0 0]  TranslationROffset=0  TranslationROffsetUnits=m  TranslationZOffset=0  TranslationZOffsetUnits=m  TranslationThetaOffset=0  TranslationThetaOffsetUnits=deg  RotationMethod=None  RotationAngleUnits=deg  RotationStandardAxis=+Z  RotationAngle=0.0  RotationArbitraryAxis=[0 0 1]  FollAlignAxisA=+X  BaseAlignAxisA=+Y  FollAlignAxisB=+Y  BaseAlignAxisB=+Z  RotationSequenceAxes=FollowerAxes  RotationSequence=XYX  RotationSequenceAngles=[0 0 0]  RotationSequenceAnglesUnits=deg  RotationMatrix=[1 0 0; 0 1 0; 0 0 1]
  CS2_to_ankle : sm_lib/Frames and Transforms/Rigid Transform  TranslationMethod=Cartesian  TranslationStandardOffset=0  TranslationLengthUnit=m  TranslationStandardAxis=+Z  TranslationCartesianOffset=[-D12_F ankle_height 0]  TranslationROffset=0  TranslationROffsetUnits=m  TranslationZOffset=0  TranslationZOffsetUnits=m  TranslationThetaOffset=0  TranslationThetaOffsetUnits=deg  RotationMethod=None  RotationAngleUnits=deg  RotationStandardAxis=+Z  RotationAngle=0.0  RotationArbitraryAxis=[0 0 1]  FollAlignAxisA=+X  BaseAlignAxisA=+Y  FollAlignAxisB=+Y  BaseAlignAxisB=+Z  RotationSequenceAxes=FollowerAxes  RotationSequence=XYX  RotationSequenceAngles=[0 0 0]  RotationSequenceAnglesUnits=deg  RotationMatrix=[1 0 0; 0 1 0; 0 0 1]
  CS3 : sm_lib/Frames and Transforms/Rigid Transform  TranslationMethod=Cartesian  TranslationStandardOffset=0  TranslationLengthUnit=m  TranslationStandardAxis=+Z  TranslationCartesianOffset=[0 0 d_fBall/2]  TranslationROffset=0  TranslationROffsetUnits=m  TranslationZOffset=0  TranslationZOffsetUnits=m  TranslationThetaOffset=0  TranslationThetaOffsetUnits=deg  RotationMethod=None  RotationAngleUnits=deg  RotationStandardAxis=+Z  RotationAngle=0.0  RotationArbitraryAxis=[0 0 1]  FollAlignAxisA=+X  BaseAlignAxisA=+Y  FollAlignAxisB=+Y  BaseAlignAxisB=+Z  RotationSequenceAxes=FollowerAxes  RotationSequence=XYX  RotationSequenceAngles=[0 0 0]  RotationSequenceAnglesUnits=deg  RotationMatrix=[1 0 0; 0 1 0; 0 0 1]
  CS4 : sm_lib/Frames and Transforms/Rigid Transform  TranslationMethod=Cartesian  TranslationStandardOffset=0  TranslationLengthUnit=m  TranslationStandardAxis=+Z  TranslationCartesianOffset=[0 0 -d_fBall/2]  TranslationROffset=0  TranslationROffsetUnits=m  TranslationZOffset=0  TranslationZOffsetUnits=m  TranslationThetaOffset=0  TranslationThetaOffsetUnits=deg  RotationMethod=None  RotationAngleUnits=deg  RotationStandardAxis=+Z  RotationAngle=0.0  RotationArbitraryAxis=[0 0 1]  FollAlignAxisA=+X  BaseAlignAxisA=+Y  FollAlignAxisB=+Y  BaseAlignAxisB=+Z  RotationSequenceAxes=FollowerAxes  RotationSequence=XYX  RotationSequenceAngles=[0 0 0]  RotationSequenceAnglesUnits=deg  RotationMatrix=[1 0 0; 0 1 0; 0 0 1]
  CS7 : sm_lib/Frames and Transforms/Rigid Transform  TranslationMethod=Cartesian  TranslationStandardOffset=0  TranslationLengthUnit=m  TranslationStandardAxis=+Z  TranslationCartesianOffset=[-D13_F 0 d_fHeel/2]  TranslationROffset=0  TranslationROffsetUnits=m  TranslationZOffset=0  TranslationZOffsetUnits=m  TranslationThetaOffset=0  TranslationThetaOffsetUnits=deg  RotationMethod=None  RotationAngleUnits=deg  RotationStandardAxis=+Z  RotationAngle=0.0  RotationArbitraryAxis=[0 0 1]  FollAlignAxisA=+X  BaseAlignAxisA=+Y  FollAlignAxisB=+Y  BaseAlignAxisB=+Z  RotationSequenceAxes=FollowerAxes  RotationSequence=XYX  RotationSequenceAngles=[0 0 0]  RotationSequenceAnglesUnits=deg  RotationMatrix=[1 0 0; 0 1 0; 0 0 1]
  CS8 : sm_lib/Frames and Transforms/Rigid Transform  TranslationMethod=Cartesian  TranslationStandardOffset=0  TranslationLengthUnit=m  TranslationStandardAxis=+Z  TranslationCartesianOffset=[-D13_F 0 -d_fHeel/2]  TranslationROffset=0  TranslationROffsetUnits=m  TranslationZOffset=0  TranslationZOffsetUnits=m  TranslationThetaOffset=0  TranslationThetaOffsetUnits=deg  RotationMethod=None  RotationAngleUnits=deg  RotationStandardAxis=+Z  RotationAngle=0.0  RotationArbitraryAxis=[0 0 1]  FollAlignAxisA=+X  BaseAlignAxisA=+Y  FollAlignAxisB=+Y  BaseAlignAxisB=+Z  RotationSequenceAxes=FollowerAxes  RotationSequence=XYX  RotationSequenceAngles=[0 0 0]  RotationSequenceAnglesUnits=deg  RotationMatrix=[1 0 0; 0 1 0; 0 0 1]
  Inertia : sm_lib/Body Elements/Inertia  InertiaType=Custom  Mass=m_F  MassUnits=kg  CenterOfMass=[0 0 0]  CenterOfMassUnits=m  MomentsOfInertia=[Inx_F Iny_F In_F]  MomentsOfInertiaUnits=kg*m^2  ProductsOfInertia=[0 0 0]  ProductsOfInertiaUnits=kg*m^2  GraphicType=None  MarkerShape=Inertia  MarkerSize=20  GraphicVisPropType=SimpleVisualProperties  GraphicDiffuseColor=[0.5 0.5 0.5]  GraphicSpecularColor=[0.5 0.5 0.5 1.0]  GraphicAmbientColor=[0.15 0.15 0.15 1.0]  GraphicEmissiveColor=[0.0 0.0 0.0 1.0]  GraphicShininess=75  GraphicOpacity=1.0
  Mux{,1..4} (5 alike) : Mux  Inputs=3
  PS-Simulink Converter{,1..14} (15 alike) : nesl_utility/PS-Simulink Converter  PhysicalDomain=network_engine_domain  SubClassName=ps_output  LeftPortType=input  RightPortType=output  PseudoPeriodic=off  Frequencies=[]  Unit=m  AffineConversion=off
  Reference Frame : sm_lib/Frames and Transforms/Reference Frame
  TO: X-forward Y-up Z-lateral : sm_lib/Frames and Transforms/Rigid Transform  TranslationMethod=StandardAxis  TranslationStandardOffset=D12z_T/2  TranslationLengthUnit=m  TranslationStandardAxis=+Y  TranslationCartesianOffset=[0 0 0]  TranslationROffset=0  TranslationROffsetUnits=m  TranslationZOffset=0  TranslationZOffsetUnits=m  TranslationThetaOffset=0  TranslationThetaOffsetUnits=deg  RotationMethod=AlignedAxes  RotationAngleUnits=deg  RotationStandardAxis=+Z  RotationAngle=0  RotationArbitraryAxis=[0 0 1]  FollAlignAxisA=+Z  BaseAlignAxisA=-Y  FollAlignAxisB=+X  BaseAlignAxisB=+X  RotationSequenceAxes=FollowerAxes  RotationSequence=XYX  RotationSequenceAngles=[0 0 0]  RotationSequenceAnglesUnits=deg  RotationMatrix=[1 0 0; 0 1 0; 0 0 1]
  To CG : sm_lib/Frames and Transforms/Rigid Transform  TranslationMethod=Cartesian  TranslationStandardOffset=0  TranslationLengthUnit=m  TranslationStandardAxis=+Z  TranslationCartesianOffset=[-D1G_F D1Gy_F 0]  TranslationROffset=0  TranslationROffsetUnits=m  TranslationZOffset=0  TranslationZOffsetUnits=m  TranslationThetaOffset=0  TranslationThetaOffsetUnits=deg  RotationMethod=None  RotationAngleUnits=deg  RotationStandardAxis=+Z  RotationAngle=0.0  RotationArbitraryAxis=[0 0 1]  FollAlignAxisA=+X  BaseAlignAxisA=+Y  FollAlignAxisB=+Y  BaseAlignAxisB=+Z  RotationSequenceAxes=FollowerAxes  RotationSequence=XYX  RotationSequenceAngles=[0 0 0]  RotationSequenceAnglesUnits=deg  RotationMatrix=[1 0 0; 0 1 0; 0 0 1]
  To center : sm_lib/Frames and Transforms/Rigid Transform  TranslationMethod=Cartesian  TranslationStandardOffset=0  TranslationLengthUnit=m  TranslationStandardAxis=+Z  TranslationCartesianOffset=[-D13_F/2 ankle_height/2 0]  TranslationROffset=0  TranslationROffsetUnits=m  TranslationZOffset=0  TranslationZOffsetUnits=m  TranslationThetaOffset=0  TranslationThetaOffsetUnits=deg  RotationMethod=None  RotationAngleUnits=deg  RotationStandardAxis=+Z  RotationAngle=0.0  RotationArbitraryAxis=[0 0 1]  FollAlignAxisA=+X  BaseAlignAxisA=+Y  FollAlignAxisB=+Y  BaseAlignAxisB=+Z  RotationSequenceAxes=FollowerAxes  RotationSequence=XYX  RotationSequenceAngles=[0 0 0]  RotationSequenceAnglesUnits=deg  RotationMatrix=[1 0 0; 0 1 0; 0 0 1]
  Transform Sensor{,1..4} (5 alike) : sm_lib/Frames and Transforms/Transform Sensor  MeasurementFrame=NonRotatingBase  SenseAngle=off  SenseAxis=off  SenseAngle1=off  SenseAngle2=off  SenseAngle3=off  SenseQ=off  SenseR=off  SenseOmegaX=off  SenseOmegaY=off  SenseOmegaZ=off  SenseOmega1=off  SenseOmega2=off  SenseOmega3=off  SenseQDot=off  SenseRDot=off  SenseAlphaX=off  SenseAlphaY=off  SenseAlphaZ=off  SenseAlpha1=off  SenseAlpha2=off  SenseAlpha3=off  SenseQDDot=off  SenseRDDot=off  SenseX=on  SenseY=on  SenseZ=on  SenseRad=off  SenseAzim=off  SenseDist=off  SenseInc=off  SenseXDot=off  SenseYDot=off  SenseZDot=off  SenseRadDot=off  SenseAzimDot=off  SenseDistDot=off  SenseIncDot=off  SenseXDDot=off  SenseYDDot=off  SenseZDDot=off  SenseRadDDot=off  SenseAzimDDot=off  SenseDistDDot=off  SenseIncDDot=off
  World Frame : sm_lib/Frames and Transforms/World Frame
  ankle : PMIOPort  Side=Right
  LLHeel Cnt : PMIOPort  Port=2  Side=Left
  LMHeel Cnt : PMIOPort  Port=3  Side=Left
  LMBall Cnt : PMIOPort  Port=4  Side=Left
  LLBall Cnt : PMIOPort  Port=5  Side=Left
  World : PMIOPort  Port=6  Side=Left
  LMBall Cnt pos : Outport
  LLBall Cnt pos : Outport  Port=2
  LMHeel Cnt pos : Outport  Port=3
  LLHeel Cnt pos : Outport  Port=4
  CG pos : Outport  Port=5
  wires:
  PS-Simulink Converter/1 -> Mux/1
  PS-Simulink Converter2/1 -> Mux/2
  PS-Simulink Converter1/1 -> Mux/3
  Mux/1 -> LMBall Cnt pos/1
  Mux1/1 -> LLBall Cnt pos/1
  PS-Simulink Converter6/1 -> Mux2/3
  Mux2/1 -> LMHeel Cnt pos/1
  PS-Simulink Converter11/1 -> Mux3/1
  Mux3/1 -> LLHeel Cnt pos/1
  PS-Simulink Converter10/1 -> Mux3/2
  PS-Simulink Converter9/1 -> Mux3/3
  PS-Simulink Converter8/1 -> Mux2/1
  PS-Simulink Converter7/1 -> Mux2/2
  PS-Simulink Converter3/1 -> Mux1/1
  PS-Simulink Converter4/1 -> Mux1/2
  PS-Simulink Converter5/1 -> Mux1/3
  PS-Simulink Converter12/1 -> Mux4/1
  PS-Simulink Converter13/1 -> Mux4/2
  PS-Simulink Converter14/1 -> Mux4/3
  Mux4/1 -> CG pos/1
  connections:
  CS5/LConn1 -- Transform Sensor1/RConn1 -- CS4/RConn1
  CS6/LConn1 -- Transform Sensor/RConn1 -- CS3/RConn1
  CS9/LConn1 -- Transform Sensor3/RConn1 -- CS8/RConn1
  CS10/LConn1 -- Transform Sensor2/RConn1 -- CS7/RConn1
  LMBall Cnt/RConn1 -- CS6/RConn1
  LLHeel Cnt/RConn1 -- CS9/RConn1
  ankle/RConn1 -- CS2_to_ankle/RConn1
  LLBall Cnt/RConn1 -- CS5/RConn1
  LMHeel Cnt/RConn1 -- CS10/RConn1
  To CG/RConn1 -- Transform Sensor4/RConn1 -- Inertia/RConn1
  World/RConn1 -- CS1/LConn1
  PS-Simulink Converter/LConn1 -- Transform Sensor/RConn2
  Transform Sensor/RConn3 -- PS-Simulink Converter2/LConn1
  Transform Sensor/RConn4 -- PS-Simulink Converter1/LConn1
  Transform Sensor2/RConn2 -- PS-Simulink Converter8/LConn1
  Transform Sensor3/RConn4 -- PS-Simulink Converter9/LConn1
  Transform Sensor2/RConn4 -- PS-Simulink Converter6/LConn1
  Transform Sensor3/RConn2 -- PS-Simulink Converter11/LConn1
  Transform Sensor2/RConn3 -- PS-Simulink Converter7/LConn1
  Transform Sensor3/RConn3 -- PS-Simulink Converter10/LConn1
  To CG/LConn1 -- CS1/RConn1 -- To center/LConn1 -- CS3/LConn1 -- CS2_to_ankle/LConn1 -- CS4/LConn1 -- CS8/LConn1 -- CS7/LConn1
  PS-Simulink Converter3/LConn1 -- Transform Sensor1/RConn2
  PS-Simulink Converter4/LConn1 -- Transform Sensor1/RConn3
  PS-Simulink Converter5/LConn1 -- Transform Sensor1/RConn4
  Brick Solid/RConn1 -- To center/RConn1
  Transform Sensor2/LConn1 -- Transform Sensor4/LConn1 -- Transform Sensor/LConn1 -- Transform Sensor1/LConn1 -- Reference Frame/RConn1 -- TO: X-forward Y-up Z-lateral/RConn1 -- Transform Sensor3/LConn1
  TO: X-forward Y-up Z-lateral/LConn1 -- World Frame/RConn1
  PS-Simulink Converter12/LConn1 -- Transform Sensor4/RConn2
  PS-Simulink Converter13/LConn1 -- Transform Sensor4/RConn3
  PS-Simulink Converter14/LConn1 -- Transform Sensor4/RConn4
